simulink model "reactor"  (R2024a)
settings: Solver=ode15s  StartTime=0.0  StopTime=420*60
model workspace (MAT data in the model file):
  ratio1 = 0.5
libraries: slident x30, slpidlib x6
settings Model: Creator=kong0225  LastModifiedBy=kong0225
settings SolverCC: ZeroCrossControl=DisableAll  ZeroCrossAlgorithm=Adaptive  SolverResetMethod=Robust
settings DataIOCC: SaveState=on
settings DebuggingCC: UnconnectedInputMsg=warning  UnconnectedOutputMsg=warning  UnconnectedLineMsg=warning
settings ModelReferenceCC: EnableRefExpFcnMdlSchedulingChecks=on  ModelReferenceMinAlgLoopOccurrences=on
settings RTWCC: GPUComputeCapability=3.5  DLArmComputeVersion=19.05

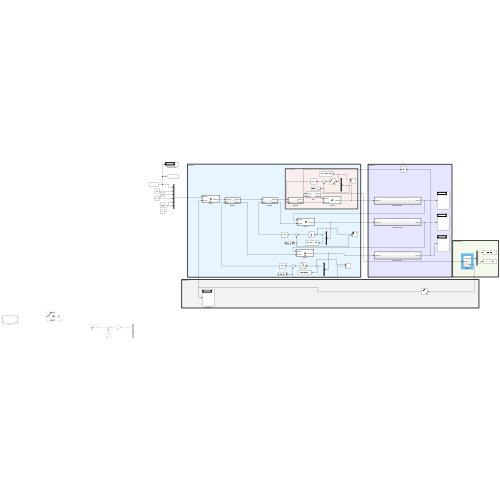
[thumbnail: Simulink's stored preview of the top-level diagram]
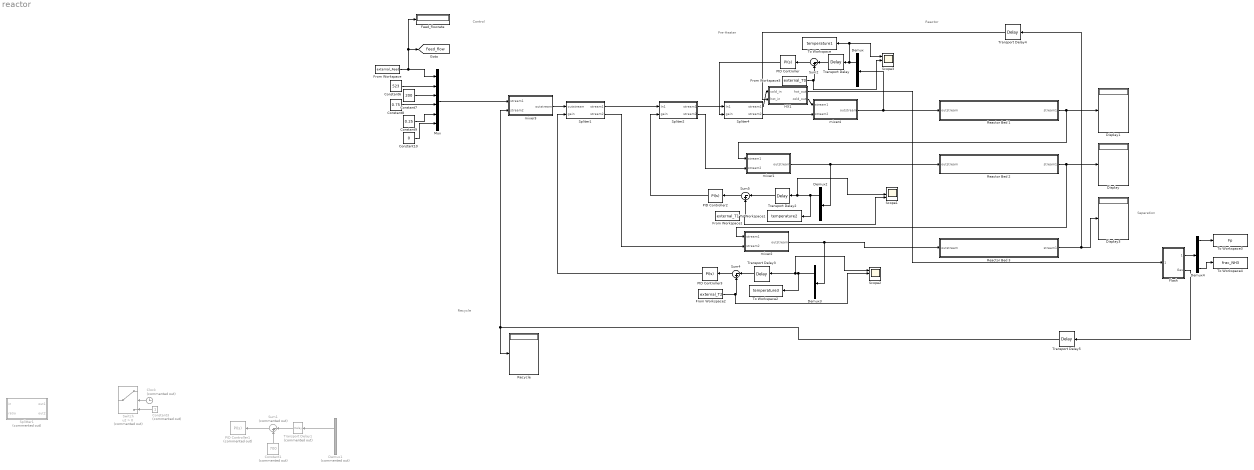
== system reactor ==
  note: Pre-Heater
  note: Control
  note: Separation
  note: Reactor
  note: Recycle
  Clock : Clock  Commented=on
  Constant1 : Constant  Commented=on  Value=700
  Constant10 : Constant  Value=0
  Constant3 : Constant  Commented=on
  Constant6 : Constant  Value=523
  Constant7 : Constant  Value=200
  Constant8 : Constant  Value=0.75
  Constant9 : Constant  Value=0.25
  Demux{,2..4} (4 alike) : Demux  Outputs=6
  Demux1 : Demux  Commented=on  Outputs=6
  Display : Display
  Display1 : Display
  Display3 : Display
  Feed_flowrate : Display
  Flash : Subsystem
  From Workspace : FromWorkspace  VariableName=external_Feed  Interpolate=off  OutputAfterFinalValue=Holding final value
  From Workspace1 : FromWorkspace  VariableName=external_T1  Interpolate=off  OutputAfterFinalValue=Holding final value
  From Workspace2 : FromWorkspace  VariableName=external_T2  Interpolate=off  OutputAfterFinalValue=Holding final value
  From Workspace3 : FromWorkspace  VariableName=external_T0  Interpolate=off  OutputAfterFinalValue=Holding final value
  HX1 : Subsystem
  Mux : Mux  Inputs=6
  PID Controller : slpidlib/PID Controller  Controller=PI  Form=Parallel  TimeDomain=Continuous-time  UseExternalTs=off  SampleTime=1  IntegratorMethod=Forward Euler  FilterMethod=Forward Euler  ControllerParametersSource=internal  P=-0.048857  I=-0.003  UseKiTs=off  D=0  UseExternalDerivativeSource=off  N=100  UseFilter=on  TunerSelectOption=Transfer Function Based (PID Tuner App)  ZeroCross=off  InitialConditionSource=internal  InitialConditionForIntegrator=0.0001  InitialConditionForFilter=0  DifferentiatorICPrevScaledInput=0  ExternalReset=none  TrackingMode=off  Kt=1  LimitOutput=off  SatLimitsSource=internal  UpperSaturationLimit=0.99  LowerSaturationLimit=-0.99  LinearizeAsGain=off  AntiWindupMode=clamping  Kb=1  LimitIntegrator=off  UpperIntegratorSaturationLimit=inf  LowerIntegratorSaturationLimit=-inf  POutMin=[]  POutMax=[]  IOutMin=[]  IOutMax=[]  DOutMin=[]  DOutMax=[]  NOutMin=[]  NOutMax=[]  SumOutMin=[]  SumOutMax=[]  SaturationOutMin=[]  SaturationOutMax=[]  PParamMin=[]  PParamMax=[]  IParamMin=[]  IParamMax=[]  DParamMin=[]  DParamMax=[]  NParamMin=[]  NParamMax=[]  KbParamMin=[]  KbParamMax=[]  KtParamMin=[]  KtParamMax=[]  KbOutMin=[]  KbOutMax=[]  KtOutMin=[]  KtOutMax=[]  IntegratorOutMin=[]  IntegratorOutMax=[]  FilterOutMin=[]  FilterOutMax=[]  SumI1OutMin=[]  SumI1OutMax=[]  SumI2OutMin=[]  SumI2OutMax=[]  SumI3OutMin=[]  SumI3OutMax=[]  SumI4OutMin=[]  SumI4OutMax=[]  SumDOutMin=[]  SumDOutMax=[]  DifferentiatorOutMin=[]  DifferentiatorOutMax=[]  FilterDiffOutCoefMin=[]  FilterDiffOutCoefMax=[]  ReciprocalOutMin=[]  ReciprocalOutMax=[]  SumDenOutMin=[]  SumDenOutMax=[]  SumNumOutMin=[]  SumNumOutMax=[]  DivideOutMin=[]  DivideOutMax=[]  UdiffTsProdOutMin=[]  UdiffTsProdOutMax=[]  NTsProdOutMin=[]  NTsProdOutMax=[]  UintegralTsProdOutMin=[]  UintegralTsProdOutMax=[]  UngainTsProdOutMin=[]  UngainTsProdOutMax=[]  ClampingZeroOutDataTypeStr=Inherit: Inherit via back propagation  ClampingZeroOutMin=[]  ClampingZeroOutMax=[]  FilterDenConstantOutDataTypeStr=Inherit: Inherit via back propagation  FilterDenConstantOutMin=[]  FilterDenConstantOutMax=[]  PCopyOutDataTypeStr=Inherit: Inherit via back propagation  PCopyOutMin=[]  PCopyOutMax=[]  NCopyOutDataTypeStr=Inherit: Inherit via back propagation  NCopyOutMin=[]  NCopyOutMax=[]  IntegratorContinuousStateAttributes=''  IntegratorStateMustResolveToSignalObject=off  IntegratorRTWStateStorageClass=Auto  FilterContinuousStateAttributes=''  FilterStateMustResolveToSignalObject=off  FilterRTWStateStorageClass=Auto  ParallelPVariant=InternalParameters  IdealPVariant=Disabled  IVariant=InternalParameters  DVariant=Disabled  IntegratorVariant=Continuous  SatVariant=Disabled  AWVariant=Passthrough  PCopyVariant=Disabled  TRVariant=Disabled  FdbkBlocksVariant=Forward  IdealPFdbkVariant=Disabled  SatFdbkVariant=Disabled  DerivativeFilterVariant=Disabled  NVariant=Disabled  NCopyVariant=Disabled_SignalSpec  FilterICVariant=Disabled  IntegratorICVariant=InternalICs  ExternalResetVariant=Disabled  TRSumVariant=Passthrough  SumFdbkVariant=Disabled  SumVariant=Sum_PI  TsampFilterVariant=InternalTs  TsampNgainVariant=Passthrough  TsampIntegralVariant=Disabled_SignalSpec  ExternalSaturationOutDataTypeStr=Inherit: Same as second input  DerivativeSourceVariant=Disabled
  PID Controller1 : slpidlib/PID Controller  Commented=on  Controller=PI  Form=Parallel  TimeDomain=Continuous-time  UseExternalTs=off  SampleTime=-1  IntegratorMethod=Forward Euler  FilterMethod=Forward Euler  ControllerParametersSource=internal  P=0.000672330279785906  I=0.00572696013263411  UseKiTs=off  D=0  UseExternalDerivativeSource=off  N=100  UseFilter=on  TunerSelectOption=Transfer Function Based (PID Tuner App)  InitialConditionSource=internal  InitialConditionForIntegrator=0  InitialConditionForFilter=0  DifferentiatorICPrevScaledInput=0  ExternalReset=none  TrackingMode=off  Kt=1  LimitOutput=on  SatLimitsSource=internal  UpperSaturationLimit=0.99  LowerSaturationLimit=0.01  LinearizeAsGain=off  AntiWindupMode=clamping  Kb=1  LimitIntegrator=off  UpperIntegratorSaturationLimit=inf  LowerIntegratorSaturationLimit=-inf  POutMin=[]  POutMax=[]  IOutMin=[]  IOutMax=[]  DOutMin=[]  DOutMax=[]  NOutMin=[]  NOutMax=[]  SumOutMin=[]  SumOutMax=[]  SaturationOutMin=[]  SaturationOutMax=[]  PParamMin=[]  PParamMax=[]  IParamMin=[]  IParamMax=[]  DParamMin=[]  DParamMax=[]  NParamMin=[]  NParamMax=[]  KbParamMin=[]  KbParamMax=[]  KtParamMin=[]  KtParamMax=[]  KbOutMin=[]  KbOutMax=[]  KtOutMin=[]  KtOutMax=[]  IntegratorOutMin=[]  IntegratorOutMax=[]  FilterOutMin=[]  FilterOutMax=[]  SumI1OutMin=[]  SumI1OutMax=[]  SumI2OutMin=[]  SumI2OutMax=[]  SumI3OutMin=[]  SumI3OutMax=[]  SumI4OutMin=[]  SumI4OutMax=[]  SumDOutMin=[]  SumDOutMax=[]  DifferentiatorOutMin=[]  DifferentiatorOutMax=[]  FilterDiffOutCoefMin=[]  FilterDiffOutCoefMax=[]  ReciprocalOutMin=[]  ReciprocalOutMax=[]  SumDenOutMin=[]  SumDenOutMax=[]  SumNumOutMin=[]  SumNumOutMax=[]  DivideOutMin=[]  DivideOutMax=[]  UdiffTsProdOutMin=[]  UdiffTsProdOutMax=[]  NTsProdOutMin=[]  NTsProdOutMax=[]  UintegralTsProdOutMin=[]  UintegralTsProdOutMax=[]  UngainTsProdOutMin=[]  UngainTsProdOutMax=[]  ClampingZeroOutDataTypeStr=Inherit: Inherit via back propagation  ClampingZeroOutMin=[]  ClampingZeroOutMax=[]  FilterDenConstantOutDataTypeStr=Inherit: Inherit via back propagation  FilterDenConstantOutMin=[]  FilterDenConstantOutMax=[]  PCopyOutDataTypeStr=Inherit: Inherit via back propagation  PCopyOutMin=[]  PCopyOutMax=[]  NCopyOutDataTypeStr=Inherit: Inherit via back propagation  NCopyOutMin=[]  NCopyOutMax=[]  IntegratorContinuousStateAttributes=''  IntegratorStateMustResolveToSignalObject=off  IntegratorRTWStateStorageClass=Auto  FilterContinuousStateAttributes=''  FilterStateMustResolveToSignalObject=off  FilterRTWStateStorageClass=Auto  ParallelPVariant=InternalParameters  IdealPVariant=Disabled  IVariant=InternalParameters  DVariant=Disabled  IntegratorVariant=Continuous  SatVariant=Enabled  AWVariant=ContClampingParallel  PCopyVariant=Disabled  TRVariant=Disabled  FdbkBlocksVariant=Forward  IdealPFdbkVariant=Disabled  SatFdbkVariant=Disabled  DerivativeFilterVariant=Disabled  NVariant=Disabled  NCopyVariant=Disabled_SignalSpec  FilterICVariant=Disabled  IntegratorICVariant=InternalICs  ExternalResetVariant=Disabled  TRSumVariant=Passthrough  SumFdbkVariant=Disabled  SumVariant=Sum_PI  TsampFilterVariant=InternalTs  TsampNgainVariant=Passthrough  TsampIntegralVariant=Passthrough  ExternalSaturationOutDataTypeStr=Inherit: Same as second input  DerivativeSourceVariant=ErrorSignal
  PID Controller2 : slpidlib/PID Controller  Controller=PI  Form=Parallel  TimeDomain=Continuous-time  UseExternalTs=off  SampleTime=1  IntegratorMethod=Forward Euler  FilterMethod=Forward Euler  ControllerParametersSource=internal  P=-0.0439115523106535  I=-0.057875624067586  UseKiTs=off  D=0  UseExternalDerivativeSource=off  N=100  UseFilter=on  TunerSelectOption=Transfer Function Based (PID Tuner App)  ZeroCross=off  InitialConditionSource=internal  InitialConditionForIntegrator=0.0001  InitialConditionForFilter=0  DifferentiatorICPrevScaledInput=0  ExternalReset=none  TrackingMode=off  Kt=1  LimitOutput=off  SatLimitsSource=internal  UpperSaturationLimit=0.99  LowerSaturationLimit=-0.99  LinearizeAsGain=off  AntiWindupMode=clamping  Kb=1  LimitIntegrator=off  UpperIntegratorSaturationLimit=inf  LowerIntegratorSaturationLimit=-inf  POutMin=[]  POutMax=[]  IOutMin=[]  IOutMax=[]  DOutMin=[]  DOutMax=[]  NOutMin=[]  NOutMax=[]  SumOutMin=[]  SumOutMax=[]  SaturationOutMin=[]  SaturationOutMax=[]  PParamMin=[]  PParamMax=[]  IParamMin=[]  IParamMax=[]  DParamMin=[]  DParamMax=[]  NParamMin=[]  NParamMax=[]  KbParamMin=[]  KbParamMax=[]  KtParamMin=[]  KtParamMax=[]  KbOutMin=[]  KbOutMax=[]  KtOutMin=[]  KtOutMax=[]  IntegratorOutMin=[]  IntegratorOutMax=[]  FilterOutMin=[]  FilterOutMax=[]  SumI1OutMin=[]  SumI1OutMax=[]  SumI2OutMin=[]  SumI2OutMax=[]  SumI3OutMin=[]  SumI3OutMax=[]  SumI4OutMin=[]  SumI4OutMax=[]  SumDOutMin=[]  SumDOutMax=[]  DifferentiatorOutMin=[]  DifferentiatorOutMax=[]  FilterDiffOutCoefMin=[]  FilterDiffOutCoefMax=[]  ReciprocalOutMin=[]  ReciprocalOutMax=[]  SumDenOutMin=[]  SumDenOutMax=[]  SumNumOutMin=[]  SumNumOutMax=[]  DivideOutMin=[]  DivideOutMax=[]  UdiffTsProdOutMin=[]  UdiffTsProdOutMax=[]  NTsProdOutMin=[]  NTsProdOutMax=[]  UintegralTsProdOutMin=[]  UintegralTsProdOutMax=[]  UngainTsProdOutMin=[]  UngainTsProdOutMax=[]  ClampingZeroOutDataTypeStr=Inherit: Inherit via back propagation  ClampingZeroOutMin=[]  ClampingZeroOutMax=[]  FilterDenConstantOutDataTypeStr=Inherit: Inherit via back propagation  FilterDenConstantOutMin=[]  FilterDenConstantOutMax=[]  PCopyOutDataTypeStr=Inherit: Inherit via back propagation  PCopyOutMin=[]  PCopyOutMax=[]  NCopyOutDataTypeStr=Inherit: Inherit via back propagation  NCopyOutMin=[]  NCopyOutMax=[]  IntegratorContinuousStateAttributes=''  IntegratorStateMustResolveToSignalObject=off  IntegratorRTWStateStorageClass=Auto  FilterContinuousStateAttributes=''  FilterStateMustResolveToSignalObject=off  FilterRTWStateStorageClass=Auto  ParallelPVariant=InternalParameters  IdealPVariant=Disabled  IVariant=InternalParameters  DVariant=Disabled  IntegratorVariant=Continuous  SatVariant=Disabled  AWVariant=Passthrough  PCopyVariant=Disabled  TRVariant=Disabled  FdbkBlocksVariant=Forward  IdealPFdbkVariant=Disabled  SatFdbkVariant=Disabled  DerivativeFilterVariant=Disabled  NVariant=Disabled  NCopyVariant=Disabled_SignalSpec  FilterICVariant=Disabled  IntegratorICVariant=InternalICs  ExternalResetVariant=Disabled  TRSumVariant=Passthrough  SumFdbkVariant=Disabled  SumVariant=Sum_PI  TsampFilterVariant=InternalTs  TsampNgainVariant=Passthrough  TsampIntegralVariant=Disabled_SignalSpec  ExternalSaturationOutDataTypeStr=Inherit: Same as second input  DerivativeSourceVariant=Disabled
  PID Controller3 : slpidlib/PID Controller  Controller=PI  Form=Parallel  TimeDomain=Continuous-time  UseExternalTs=off  SampleTime=1  IntegratorMethod=Forward Euler  FilterMethod=Forward Euler  ControllerParametersSource=internal  P=-0.021226  I=-0.00084495  UseKiTs=off  D=0  UseExternalDerivativeSource=off  N=100  UseFilter=on  TunerSelectOption=Transfer Function Based (PID Tuner App)  ZeroCross=off  InitialConditionSource=internal  InitialConditionForIntegrator=0.0001  InitialConditionForFilter=0  DifferentiatorICPrevScaledInput=0  ExternalReset=none  TrackingMode=off  Kt=1  LimitOutput=off  SatLimitsSource=internal  UpperSaturationLimit=0.99  LowerSaturationLimit=-0.99  LinearizeAsGain=off  AntiWindupMode=clamping  Kb=1  LimitIntegrator=off  UpperIntegratorSaturationLimit=inf  LowerIntegratorSaturationLimit=-inf  POutMin=[]  POutMax=[]  IOutMin=[]  IOutMax=[]  DOutMin=[]  DOutMax=[]  NOutMin=[]  NOutMax=[]  SumOutMin=[]  SumOutMax=[]  SaturationOutMin=[]  SaturationOutMax=[]  PParamMin=[]  PParamMax=[]  IParamMin=[]  IParamMax=[]  DParamMin=[]  DParamMax=[]  NParamMin=[]  NParamMax=[]  KbParamMin=[]  KbParamMax=[]  KtParamMin=[]  KtParamMax=[]  KbOutMin=[]  KbOutMax=[]  KtOutMin=[]  KtOutMax=[]  IntegratorOutMin=[]  IntegratorOutMax=[]  FilterOutMin=[]  FilterOutMax=[]  SumI1OutMin=[]  SumI1OutMax=[]  SumI2OutMin=[]  SumI2OutMax=[]  SumI3OutMin=[]  SumI3OutMax=[]  SumI4OutMin=[]  SumI4OutMax=[]  SumDOutMin=[]  SumDOutMax=[]  DifferentiatorOutMin=[]  DifferentiatorOutMax=[]  FilterDiffOutCoefMin=[]  FilterDiffOutCoefMax=[]  ReciprocalOutMin=[]  ReciprocalOutMax=[]  SumDenOutMin=[]  SumDenOutMax=[]  SumNumOutMin=[]  SumNumOutMax=[]  DivideOutMin=[]  DivideOutMax=[]  UdiffTsProdOutMin=[]  UdiffTsProdOutMax=[]  NTsProdOutMin=[]  NTsProdOutMax=[]  UintegralTsProdOutMin=[]  UintegralTsProdOutMax=[]  UngainTsProdOutMin=[]  UngainTsProdOutMax=[]  ClampingZeroOutDataTypeStr=Inherit: Inherit via back propagation  ClampingZeroOutMin=[]  ClampingZeroOutMax=[]  FilterDenConstantOutDataTypeStr=Inherit: Inherit via back propagation  FilterDenConstantOutMin=[]  FilterDenConstantOutMax=[]  PCopyOutDataTypeStr=Inherit: Inherit via back propagation  PCopyOutMin=[]  PCopyOutMax=[]  NCopyOutDataTypeStr=Inherit: Inherit via back propagation  NCopyOutMin=[]  NCopyOutMax=[]  IntegratorContinuousStateAttributes=''  IntegratorStateMustResolveToSignalObject=off  IntegratorRTWStateStorageClass=Auto  FilterContinuousStateAttributes=''  FilterStateMustResolveToSignalObject=off  FilterRTWStateStorageClass=Auto  ParallelPVariant=InternalParameters  IdealPVariant=Disabled  IVariant=InternalParameters  DVariant=Disabled  IntegratorVariant=Continuous  SatVariant=Disabled  AWVariant=Passthrough  PCopyVariant=Disabled  TRVariant=Disabled  FdbkBlocksVariant=Forward  IdealPFdbkVariant=Disabled  SatFdbkVariant=Disabled  DerivativeFilterVariant=Disabled  NVariant=Disabled  NCopyVariant=Disabled_SignalSpec  FilterICVariant=Disabled  IntegratorICVariant=InternalICs  ExternalResetVariant=Disabled  TRSumVariant=Passthrough  SumFdbkVariant=Disabled  SumVariant=Sum_PI  TsampFilterVariant=InternalTs  TsampNgainVariant=Passthrough  TsampIntegralVariant=Disabled_SignalSpec  ExternalSaturationOutDataTypeStr=Inherit: Same as second input  DerivativeSourceVariant=Disabled
  Reactor Bed 1 : Subsystem  TreatAsAtomicUnit=on
  Reactor Bed 2 : Subsystem  TreatAsAtomicUnit=on
  Reactor Bed 3 : Subsystem  TreatAsAtomicUnit=on
  Recycle : Display
  Scope1 : Scope  NumInputPorts=3
  Scope2 : Scope  NumInputPorts=3
  Scope3 : Scope  NumInputPorts=3
  Spliter1 : Subsystem  TreatAsAtomicUnit=on
  Spliter2 : Subsystem  TreatAsAtomicUnit=on
  Spliter4 : Subsystem  TreatAsAtomicUnit=on
  Splitter1 : MATLAB Function  Commented=on  TreatAsAtomicUnit=on
  Sum1 : Sum  Commented=on  Inputs=|-+
  Sum2 : Sum  Inputs=|-+
  Sum4 : Sum  Inputs=|-+
  Sum5 : Sum  Inputs=|-+
  Switch : Switch  Commented=on  Criteria=u2 > Threshold  SaturateOnIntegerOverflow=off  InputSameDT=off
  To Workspace : ToWorkspace  VariableName=temperature1  SaveFormat=Timeseries  SampleTime=-1
  To Workspace1 : ToWorkspace  VariableName=temperature2  SaveFormat=Timeseries  SampleTime=-1
  To Workspace2 : ToWorkspace  VariableName=temperature3  SaveFormat=Timeseries  SampleTime=-1
  To Workspace3 : ToWorkspace  VariableName=Fp  SaveFormat=Timeseries  SampleTime=-1
  To Workspace4 : ToWorkspace  VariableName=frac_NH3  SaveFormat=Timeseries  SampleTime=-1
  Transport Delay : TransportDelay  InitialOutput=635
  Transport Delay1 : TransportDelay  Commented=on  InitialOutput=700
  Transport Delay2 : TransportDelay  InitialOutput=635
  Transport Delay3 : TransportDelay  InitialOutput=635
  Transport Delay4 : TransportDelay  InitialOutput=[1500;726;200;0.6;0.2;0.2]
  Transport Delay5 : TransportDelay  InitialOutput=[2100;523;200;0.75;.25;0]
  mixer1 : MATLAB Function  TreatAsAtomicUnit=on
  mixer2 : MATLAB Function  TreatAsAtomicUnit=on
  mixer3 : MATLAB Function  TreatAsAtomicUnit=on
  mixer4 : MATLAB Function  TreatAsAtomicUnit=on
  tag scope: Feed_flow=global
  wires:
  Constant1/1 -> Sum1/2
  Demux1/2 -> Transport Delay1/1
  Transport Delay1/1 -> Sum1/1
  Clock/1 -> Switch/2
  Constant3/1 -> Switch/3
  Sum1/1 -> PID Controller1/1
  Constant6/1 -> Mux/2
  Constant7/1 -> Mux/3
  Constant8/1 -> Mux/4
  Constant9/1 -> Mux/5
  Constant10/1 -> Mux/6
  From Workspace/1 -> Feed_flowrate/1, [Feed_flow], Mux/1
  Demux3/2 -> Scope2/1, Transport Delay3/1, To Workspace2/1
  Demux2/2 -> Scope1/2, Transport Delay2/1, To Workspace1/1
  Flash/2(Gas) -> Transport Delay5/1
  Mux/1 -> mixer3/1(stream1)
  Spliter4/2(stream2) -> mixer4/2(stream2)
  Transport Delay3/1 -> Sum4/1
  HX1/2(cold_out) -> mixer4/1(stream1)
  Spliter2/1(stream1) -> Spliter4/1(In1)
  mixer1/1(outstream) -> Reactor Bed 2/1(outstream), Demux2/1
  Reactor Bed 1/1(stream1) -> mixer1/1(stream1), Display1/1
  mixer4/1(outstream) -> Reactor Bed 1/1(outstream), Demux/1
  From Workspace2/1 -> Scope2/2, Sum4/2
  Spliter1/2(stream2) -> mixer2/2(stream2)
  Reactor Bed 3/1(stream1) -> Transport Delay4/1, Display3/1
  Spliter2/2(stream2) -> mixer1/2(stream2)
  Spliter1/1(stream1) -> Spliter2/1(In1)
  Reactor Bed 2/1(stream1) -> mixer2/1(stream1), Display/1
  Transport Delay5/1 -> Recycle/1, mixer3/2(stream2)
  mixer2/1(outstream) -> Reactor Bed 3/1(outstream), Demux3/1
  Demux/2 -> Scope3/1, To Workspace/1, Transport Delay/1
  Transport Delay2/1 -> Sum5/1
  From Workspace1/1 -> Scope1/3, Sum5/2
  Spliter4/1(stream1) -> HX1/1(cold_in)
  From Workspace3/1 -> Scope3/2, Sum2/2
  HX1/1(hot_out) -> Flash/1(stream1)
  Flash/1(Ammonia) -> Demux4/1
  Demux4/1 -> To Workspace3/1
  Demux4/6 -> To Workspace4/1
  Transport Delay/1 -> Sum2/1
  Transport Delay4/1 -> HX1/2(hot_in)
  PID Controller/1 -> Spliter4/2(gain)
  Sum2/1 -> PID Controller/1
  PID Controller2/1 -> Spliter2/2(gain)
  Sum5/1 -> PID Controller2/1
  PID Controller3/1 -> Spliter1/2(gain)
  Sum4/1 -> PID Controller3/1
  mixer3/1(outstream) -> Spliter1/1(outstream)

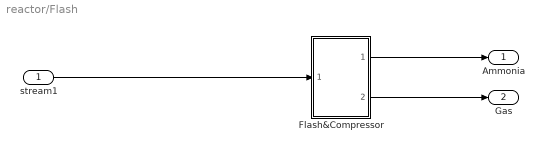
== system reactor/Flash ==
  stream1 : Inport
  Flash&Compressor : Subsystem
  Ammonia : Outport
  Gas : Outport  Port=2
  wires:
  stream1/1 -> Flash&Compressor/1(stream1)
  Flash&Compressor/1(s_prod) -> Ammonia/1
  Flash&Compressor/2(s_cyc) -> Gas/1

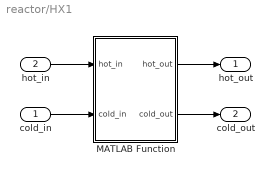
== system reactor/HX1 ==
  cold_in : Inport
  hot_in : Inport  Port=2
  MATLAB Function : MATLAB Function  TreatAsAtomicUnit=on
  hot_out : Outport
  cold_out : Outport  Port=2
  wires:
  hot_in/1 -> MATLAB Function/1(hot_in)
  cold_in/1 -> MATLAB Function/2(cold_in)
  MATLAB Function/1(hot_out) -> hot_out/1
  MATLAB Function/2(cold_out) -> cold_out/1

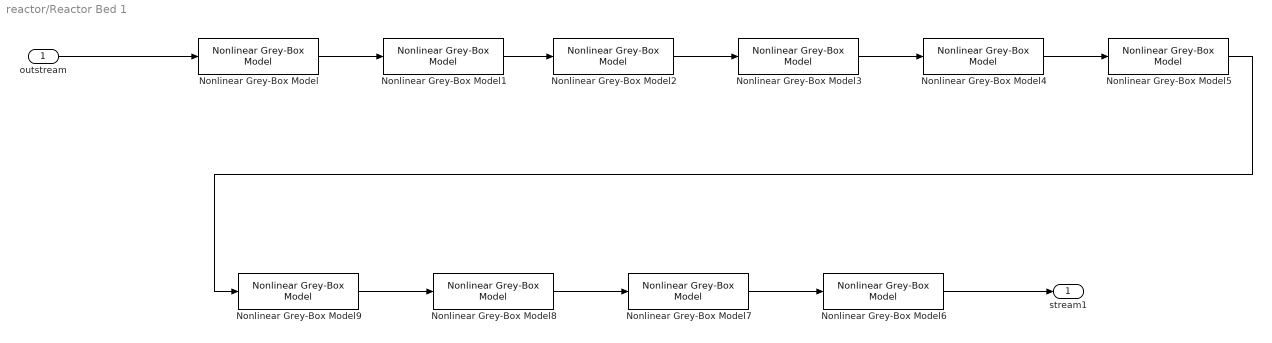
== system reactor/Reactor Bed 1 ==
  outstream : Inport
  Nonlinear Grey-Box Model : slident/Models/Nonlinear Grey-Box Model  nlsys=nlgr.nlgr_11  X0='m'
  Nonlinear Grey-Box Model1 : slident/Models/Nonlinear Grey-Box Model  nlsys=nlgr.nlgr_12  X0='m'
  Nonlinear Grey-Box Model2 : slident/Models/Nonlinear Grey-Box Model  nlsys=nlgr.nlgr_13  X0='m'
  Nonlinear Grey-Box Model3 : slident/Models/Nonlinear Grey-Box Model  nlsys=nlgr.nlgr_14  X0='m'
  Nonlinear Grey-Box Model4 : slident/Models/Nonlinear Grey-Box Model  nlsys=nlgr.nlgr_15  X0='m'
  Nonlinear Grey-Box Model5 : slident/Models/Nonlinear Grey-Box Model  nlsys=nlgr.nlgr_16  X0='m'
  Nonlinear Grey-Box Model6 : slident/Models/Nonlinear Grey-Box Model  nlsys=nlgr.nlgr_110  X0='m'
  Nonlinear Grey-Box Model7 : slident/Models/Nonlinear Grey-Box Model  nlsys=nlgr.nlgr_19  X0='m'
  Nonlinear Grey-Box Model8 : slident/Models/Nonlinear Grey-Box Model  nlsys=nlgr.nlgr_18  X0='m'
  Nonlinear Grey-Box Model9 : slident/Models/Nonlinear Grey-Box Model  nlsys=nlgr.nlgr_17  X0='m'
  stream1 : Outport
  wires:
  Nonlinear Grey-Box Model/1 -> Nonlinear Grey-Box Model1/1
  Nonlinear Grey-Box Model2/1 -> Nonlinear Grey-Box Model3/1
  Nonlinear Grey-Box Model1/1 -> Nonlinear Grey-Box Model2/1
  outstream/1 -> Nonlinear Grey-Box Model/1
  Nonlinear Grey-Box Model3/1 -> Nonlinear Grey-Box Model4/1
  Nonlinear Grey-Box Model4/1 -> Nonlinear Grey-Box Model5/1
  Nonlinear Grey-Box Model7/1 -> Nonlinear Grey-Box Model6/1
  Nonlinear Grey-Box Model8/1 -> Nonlinear Grey-Box Model7/1
  Nonlinear Grey-Box Model9/1 -> Nonlinear Grey-Box Model8/1
  Nonlinear Grey-Box Model5/1 -> Nonlinear Grey-Box Model9/1
  Nonlinear Grey-Box Model6/1 -> stream1/1

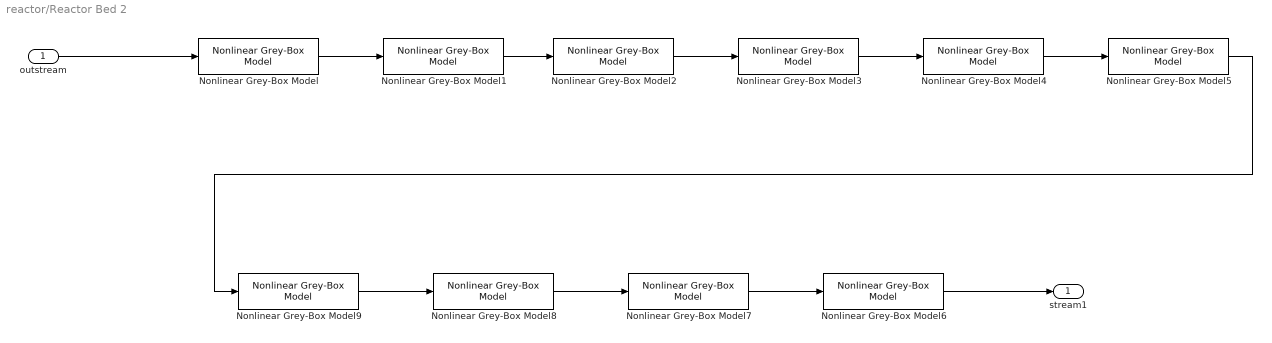
== system reactor/Reactor Bed 2 ==
  outstream : Inport
  Nonlinear Grey-Box Model : slident/Models/Nonlinear Grey-Box Model  nlsys=nlgr.nlgr_21  X0='m'
  Nonlinear Grey-Box Model1 : slident/Models/Nonlinear Grey-Box Model  nlsys=nlgr.nlgr_22  X0='m'
  Nonlinear Grey-Box Model2 : slident/Models/Nonlinear Grey-Box Model  nlsys=nlgr.nlgr_23  X0='m'
  Nonlinear Grey-Box Model3 : slident/Models/Nonlinear Grey-Box Model  nlsys=nlgr.nlgr_24  X0='m'
  Nonlinear Grey-Box Model4 : slident/Models/Nonlinear Grey-Box Model  nlsys=nlgr.nlgr_25  X0='m'
  Nonlinear Grey-Box Model5 : slident/Models/Nonlinear Grey-Box Model  nlsys=nlgr.nlgr_26  X0='m'
  Nonlinear Grey-Box Model6 : slident/Models/Nonlinear Grey-Box Model  nlsys=nlgr.nlgr_210  X0='m'
  Nonlinear Grey-Box Model7 : slident/Models/Nonlinear Grey-Box Model  nlsys=nlgr.nlgr_29  X0='m'
  Nonlinear Grey-Box Model8 : slident/Models/Nonlinear Grey-Box Model  nlsys=nlgr.nlgr_28  X0='m'
  Nonlinear Grey-Box Model9 : slident/Models/Nonlinear Grey-Box Model  nlsys=nlgr.nlgr_27  X0='m'
  stream1 : Outport
  wires:
  Nonlinear Grey-Box Model7/1 -> Nonlinear Grey-Box Model6/1
  Nonlinear Grey-Box Model9/1 -> Nonlinear Grey-Box Model8/1
  Nonlinear Grey-Box Model8/1 -> Nonlinear Grey-Box Model7/1
  Nonlinear Grey-Box Model4/1 -> Nonlinear Grey-Box Model5/1
  outstream/1 -> Nonlinear Grey-Box Model/1
  Nonlinear Grey-Box Model/1 -> Nonlinear Grey-Box Model1/1
  Nonlinear Grey-Box Model5/1 -> Nonlinear Grey-Box Model9/1
  Nonlinear Grey-Box Model1/1 -> Nonlinear Grey-Box Model2/1
  Nonlinear Grey-Box Model2/1 -> Nonlinear Grey-Box Model3/1
  Nonlinear Grey-Box Model6/1 -> stream1/1
  Nonlinear Grey-Box Model3/1 -> Nonlinear Grey-Box Model4/1

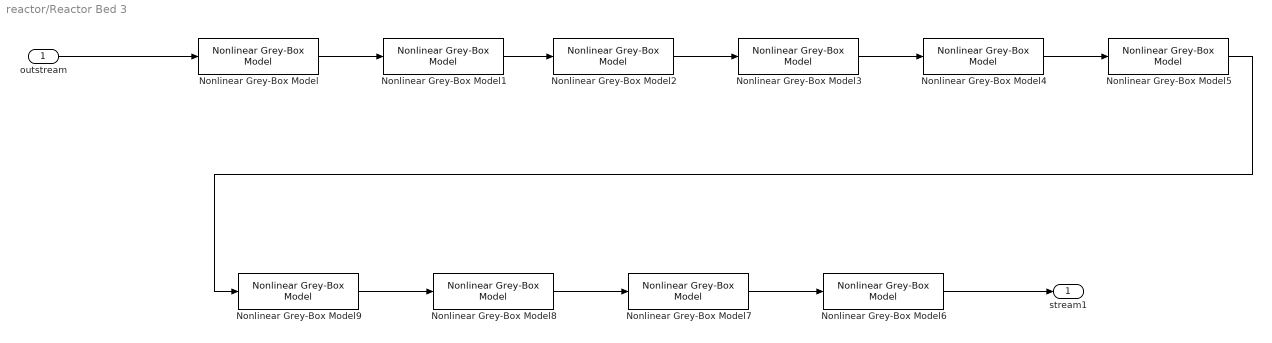
== system reactor/Reactor Bed 3 ==
  outstream : Inport
  Nonlinear Grey-Box Model : slident/Models/Nonlinear Grey-Box Model  nlsys=nlgr.nlgr_31  X0='m'
  Nonlinear Grey-Box Model1 : slident/Models/Nonlinear Grey-Box Model  nlsys=nlgr.nlgr_32  X0='m'
  Nonlinear Grey-Box Model2 : slident/Models/Nonlinear Grey-Box Model  nlsys=nlgr.nlgr_33  X0='m'
  Nonlinear Grey-Box Model3 : slident/Models/Nonlinear Grey-Box Model  nlsys=nlgr.nlgr_34  X0='m'
  Nonlinear Grey-Box Model4 : slident/Models/Nonlinear Grey-Box Model  nlsys=nlgr.nlgr_35  X0='m'
  Nonlinear Grey-Box Model5 : slident/Models/Nonlinear Grey-Box Model  nlsys=nlgr.nlgr_36  X0='m'
  Nonlinear Grey-Box Model6 : slident/Models/Nonlinear Grey-Box Model  nlsys=nlgr.nlgr_310  X0='m'
  Nonlinear Grey-Box Model7 : slident/Models/Nonlinear Grey-Box Model  nlsys=nlgr.nlgr_39  X0='m'
  Nonlinear Grey-Box Model8 : slident/Models/Nonlinear Grey-Box Model  nlsys=nlgr.nlgr_38  X0='m'
  Nonlinear Grey-Box Model9 : slident/Models/Nonlinear Grey-Box Model  nlsys=nlgr.nlgr_37  X0='m'
  stream1 : Outport
  wires:
  Nonlinear Grey-Box Model7/1 -> Nonlinear Grey-Box Model6/1
  Nonlinear Grey-Box Model9/1 -> Nonlinear Grey-Box Model8/1
  Nonlinear Grey-Box Model8/1 -> Nonlinear Grey-Box Model7/1
  Nonlinear Grey-Box Model4/1 -> Nonlinear Grey-Box Model5/1
  outstream/1 -> Nonlinear Grey-Box Model/1
  Nonlinear Grey-Box Model/1 -> Nonlinear Grey-Box Model1/1
  Nonlinear Grey-Box Model5/1 -> Nonlinear Grey-Box Model9/1
  Nonlinear Grey-Box Model1/1 -> Nonlinear Grey-Box Model2/1
  Nonlinear Grey-Box Model2/1 -> Nonlinear Grey-Box Model3/1
  Nonlinear Grey-Box Model6/1 -> stream1/1
  Nonlinear Grey-Box Model3/1 -> Nonlinear Grey-Box Model4/1

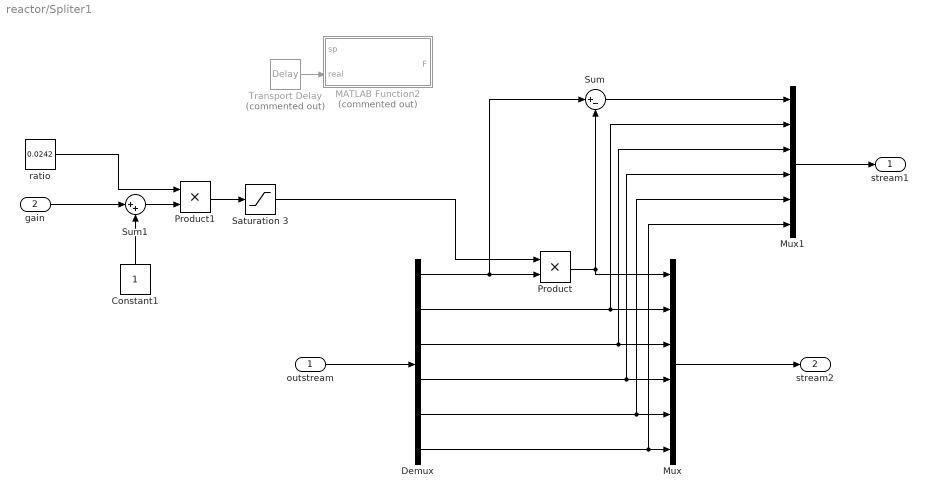
== system reactor/Spliter1 ==
  outstream : Inport
  gain : Inport  Port=2
  Constant1 : Constant
  Demux : Demux  Outputs=6
  MATLAB Function2 : MATLAB Function  Commented=on  TreatAsAtomicUnit=on
  Mux : Mux  Inputs=6
  Mux1 : Mux  Inputs=6
  Product : Product
  Product1 : Product
  Saturation 3 : Saturate  LowerLimit=0.001
  Sum : Sum  Inputs=|+-
  Sum1 : Sum  Inputs=|++
  Transport Delay : TransportDelay  Commented=on
  ratio : Constant  Value=0.0242  VectorParams1D=off
  stream1 : Outport
  stream2 : Outport  Port=2
  wires:
  outstream/1 -> Demux/1
  Demux/1 -> Sum/1, Product/2
  Product/1 -> Sum/2, Mux/1
  Demux/2 -> Mux1/2, Mux/2
  Demux/4 -> Mux1/4, Mux/4
  Demux/5 -> Mux1/5, Mux/5
  Demux/6 -> Mux1/6, Mux/6
  Sum/1 -> Mux1/1
  Demux/3 -> Mux1/3, Mux/3
  ratio/1 -> Product1/1
  gain/1 -> Sum1/1
  Constant1/1 -> Sum1/2
  Sum1/1 -> Product1/2
  Product1/1 -> Saturation 3/1
  Mux/1 -> stream2/1
  Mux1/1 -> stream1/1
  Saturation 3/1 -> Product/1
  Transport Delay/1 -> MATLAB Function2/2(real)

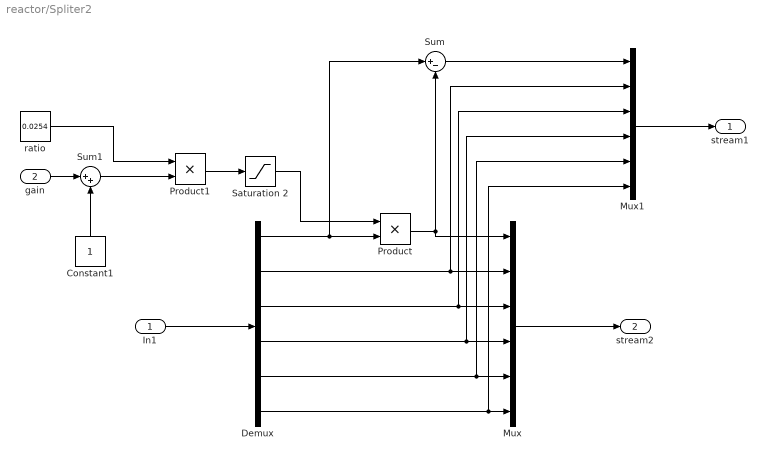
== system reactor/Spliter2 ==
  In1 : Inport
  gain : Inport  Port=2
  Constant1 : Constant
  Demux : Demux  Outputs=6
  Mux : Mux  Inputs=6
  Mux1 : Mux  Inputs=6
  Product : Product
  Product1 : Product
  Saturation 2 : Saturate  UpperLimit=0.6  LowerLimit=0.001
  Sum : Sum  Inputs=|+-
  Sum1 : Sum  Inputs=|++
  ratio : Constant  Value=0.0254
  stream1 : Outport
  stream2 : Outport  Port=2
  wires:
  In1/1 -> Demux/1
  Demux/1 -> Sum/1, Product/2
  Product/1 -> Sum/2, Mux/1
  Demux/2 -> Mux1/2, Mux/2
  Demux/4 -> Mux1/4, Mux/4
  Demux/5 -> Mux1/5, Mux/5
  Demux/6 -> Mux1/6, Mux/6
  Sum/1 -> Mux1/1
  Demux/3 -> Mux1/3, Mux/3
  Product1/1 -> Saturation 2/1
  Constant1/1 -> Sum1/2
  gain/1 -> Sum1/1
  ratio/1 -> Product1/1
  Sum1/1 -> Product1/2
  Mux/1 -> stream2/1
  Mux1/1 -> stream1/1
  Saturation 2/1 -> Product/1

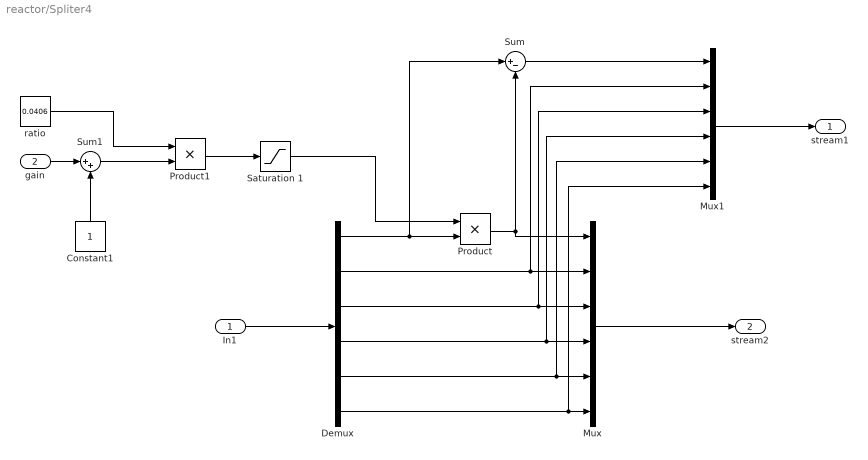
== system reactor/Spliter4 ==
  In1 : Inport
  gain : Inport  Port=2
  Constant1 : Constant
  Demux : Demux  Outputs=6
  Mux : Mux  Inputs=6
  Mux1 : Mux  Inputs=6
  Product : Product
  Product1 : Product
  Saturation 1 : Saturate  UpperLimit=0.7  LowerLimit=0.001
  Sum : Sum  Inputs=|+-
  Sum1 : Sum  Inputs=|++
  ratio : Constant  Value=0.0406
  stream1 : Outport
  stream2 : Outport  Port=2
  wires:
  In1/1 -> Demux/1
  Demux/1 -> Sum/1, Product/2
  Product/1 -> Mux/1, Sum/2
  Demux/2 -> Mux1/2, Mux/2
  Demux/4 -> Mux1/4, Mux/4
  Demux/5 -> Mux1/5, Mux/5
  Demux/6 -> Mux1/6, Mux/6
  Sum/1 -> Mux1/1
  Demux/3 -> Mux1/3, Mux/3
  Product1/1 -> Saturation 1/1
  Constant1/1 -> Sum1/2
  gain/1 -> Sum1/1
  ratio/1 -> Product1/1
  Sum1/1 -> Product1/2
  Saturation 1/1 -> Product/1
  Mux/1 -> stream2/1
  Mux1/1 -> stream1/1

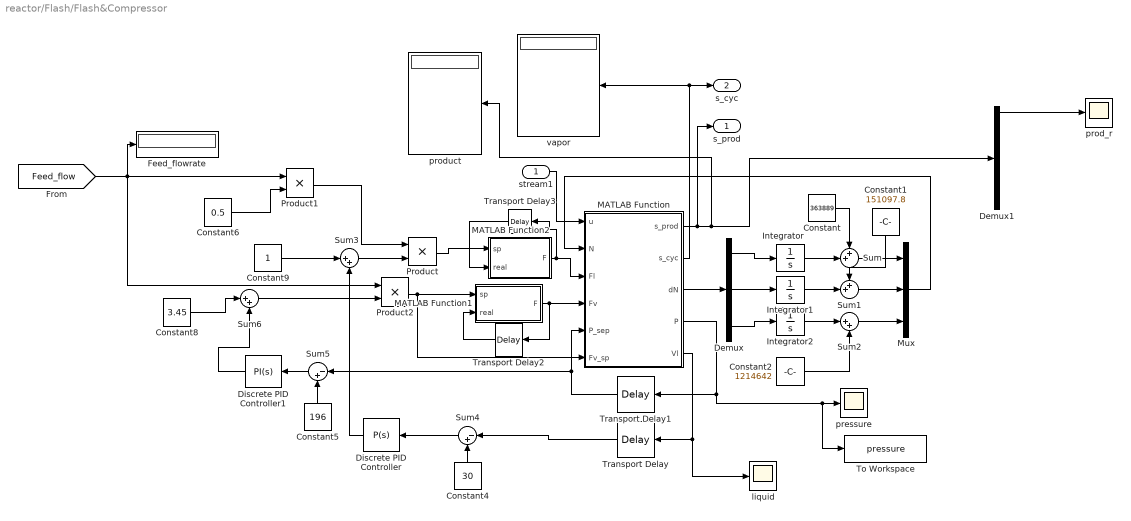
== system reactor/Flash/Flash&Compressor ==
  stream1 : Inport
  Constant : Constant  Value=363889
  Constant1 : Constant  Value=151097.8
  Constant2 : Constant  Value=1214642
  Constant4 : Constant  Value=30
  Constant5 : Constant  Value=196
  Constant6 : Constant  Value=0.5
  Constant8 : Constant  Value=3.45
  Constant9 : Constant
  Demux : Demux  Outputs=3
  Demux1 : Demux  Outputs=6
  Discrete PID Controller : slpidlib/PID Controller  Controller=P  Form=Parallel  TimeDomain=Continuous-time  UseExternalTs=off  SampleTime=-1  IntegratorMethod=Forward Euler  FilterMethod=Forward Euler  ControllerParametersSource=internal  P=-2  I=1  UseKiTs=off  D=0  UseExternalDerivativeSource=off  N=100  UseFilter=on  TunerSelectOption=Transfer Function Based (PID Tuner App)  InitialConditionSource=internal  InitialConditionForIntegrator=0  InitialConditionForFilter=0  DifferentiatorICPrevScaledInput=0  ExternalReset=none  TrackingMode=off  Kt=1  LimitOutput=on  SatLimitsSource=internal  UpperSaturationLimit=0.5  LowerSaturationLimit=-0.5  LinearizeAsGain=off  AntiWindupMode=none  Kb=1  LimitIntegrator=off  UpperIntegratorSaturationLimit=inf  LowerIntegratorSaturationLimit=-inf  POutMin=[]  POutMax=[]  IOutMin=[]  IOutMax=[]  DOutMin=[]  DOutMax=[]  NOutMin=[]  NOutMax=[]  SumOutMin=[]  SumOutMax=[]  SaturationOutMin=[]  SaturationOutMax=[]  PParamMin=[]  PParamMax=[]  IParamMin=[]  IParamMax=[]  DParamMin=[]  DParamMax=[]  NParamMin=[]  NParamMax=[]  KbParamMin=[]  KbParamMax=[]  KtParamMin=[]  KtParamMax=[]  KbOutMin=[]  KbOutMax=[]  KtOutMin=[]  KtOutMax=[]  IntegratorOutMin=[]  IntegratorOutMax=[]  FilterOutMin=[]  FilterOutMax=[]  SumI1OutMin=[]  SumI1OutMax=[]  SumI2OutMin=[]  SumI2OutMax=[]  SumI3OutMin=[]  SumI3OutMax=[]  SumI4OutMin=[]  SumI4OutMax=[]  SumDOutMin=[]  SumDOutMax=[]  DifferentiatorOutMin=[]  DifferentiatorOutMax=[]  FilterDiffOutCoefMin=[]  FilterDiffOutCoefMax=[]  ReciprocalOutMin=[]  ReciprocalOutMax=[]  SumDenOutMin=[]  SumDenOutMax=[]  SumNumOutMin=[]  SumNumOutMax=[]  DivideOutMin=[]  DivideOutMax=[]  UdiffTsProdOutMin=[]  UdiffTsProdOutMax=[]  NTsProdOutMin=[]  NTsProdOutMax=[]  UintegralTsProdOutMin=[]  UintegralTsProdOutMax=[]  UngainTsProdOutMin=[]  UngainTsProdOutMax=[]  ClampingZeroOutDataTypeStr=Inherit: Inherit via back propagation  ClampingZeroOutMin=[]  ClampingZeroOutMax=[]  FilterDenConstantOutDataTypeStr=Inherit: Inherit via back propagation  FilterDenConstantOutMin=[]  FilterDenConstantOutMax=[]  PCopyOutDataTypeStr=Inherit: Inherit via back propagation  PCopyOutMin=[]  PCopyOutMax=[]  NCopyOutDataTypeStr=Inherit: Inherit via back propagation  NCopyOutMin=[]  NCopyOutMax=[]  IntegratorContinuousStateAttributes=''  IntegratorStateMustResolveToSignalObject=off  IntegratorRTWStateStorageClass=Auto  FilterContinuousStateAttributes=''  FilterStateMustResolveToSignalObject=off  FilterRTWStateStorageClass=Auto  ParallelPVariant=InternalParameters  IdealPVariant=Disabled  IVariant=Disabled  DVariant=Disabled  IntegratorVariant=Disabled  SatVariant=Enabled  AWVariant=Disabled  PCopyVariant=Disabled  TRVariant=Disabled  FdbkBlocksVariant=Forward  IdealPFdbkVariant=Disabled  SatFdbkVariant=Disabled  DerivativeFilterVariant=Disabled  NVariant=Disabled  NCopyVariant=Disabled_SignalSpec  FilterICVariant=Disabled  IntegratorICVariant=Disabled  ExternalResetVariant=Disabled  TRSumVariant=Passthrough  SumFdbkVariant=Disabled  SumVariant=Passthrough_P  TsampFilterVariant=InternalTs  TsampNgainVariant=Passthrough  TsampIntegralVariant=Disabled_SignalSpec  ExternalSaturationOutDataTypeStr=Inherit: Same as second input  DerivativeSourceVariant=Disabled
  Discrete PID Controller1 : slpidlib/PID Controller  Controller=PI  Form=Parallel  TimeDomain=Continuous-time  UseExternalTs=off  SampleTime=-1  IntegratorMethod=Forward Euler  FilterMethod=Forward Euler  ControllerParametersSource=internal  P=-0.254  I=-0.0003  UseKiTs=off  D=-417.104440098683  UseExternalDerivativeSource=off  N=0.0199591173186702  UseFilter=on  TunerSelectOption=Transfer Function Based (PID Tuner App)  InitialConditionSource=internal  InitialConditionForIntegrator=0  InitialConditionForFilter=0  DifferentiatorICPrevScaledInput=0  ExternalReset=none  TrackingMode=off  Kt=1  LimitOutput=on  SatLimitsSource=internal  UpperSaturationLimit=1.5  LowerSaturationLimit=-1.5  LinearizeAsGain=on  AntiWindupMode=none  Kb=1  LimitIntegrator=off  UpperIntegratorSaturationLimit=inf  LowerIntegratorSaturationLimit=-inf  POutMin=[]  POutMax=[]  IOutMin=[]  IOutMax=[]  DOutMin=[]  DOutMax=[]  NOutMin=[]  NOutMax=[]  SumOutMin=[]  SumOutMax=[]  SaturationOutMin=[]  SaturationOutMax=[]  PParamMin=[]  PParamMax=[]  IParamMin=[]  IParamMax=[]  DParamMin=[]  DParamMax=[]  NParamMin=[]  NParamMax=[]  KbParamMin=[]  KbParamMax=[]  KtParamMin=[]  KtParamMax=[]  KbOutMin=[]  KbOutMax=[]  KtOutMin=[]  KtOutMax=[]  IntegratorOutMin=[]  IntegratorOutMax=[]  FilterOutMin=[]  FilterOutMax=[]  SumI1OutMin=[]  SumI1OutMax=[]  SumI2OutMin=[]  SumI2OutMax=[]  SumI3OutMin=[]  SumI3OutMax=[]  SumI4OutMin=[]  SumI4OutMax=[]  SumDOutMin=[]  SumDOutMax=[]  DifferentiatorOutMin=[]  DifferentiatorOutMax=[]  FilterDiffOutCoefMin=[]  FilterDiffOutCoefMax=[]  ReciprocalOutMin=[]  ReciprocalOutMax=[]  SumDenOutMin=[]  SumDenOutMax=[]  SumNumOutMin=[]  SumNumOutMax=[]  DivideOutMin=[]  DivideOutMax=[]  UdiffTsProdOutMin=[]  UdiffTsProdOutMax=[]  NTsProdOutMin=[]  NTsProdOutMax=[]  UintegralTsProdOutMin=[]  UintegralTsProdOutMax=[]  UngainTsProdOutMin=[]  UngainTsProdOutMax=[]  ClampingZeroOutDataTypeStr=Inherit: Inherit via back propagation  ClampingZeroOutMin=[]  ClampingZeroOutMax=[]  FilterDenConstantOutDataTypeStr=Inherit: Inherit via back propagation  FilterDenConstantOutMin=[]  FilterDenConstantOutMax=[]  PCopyOutDataTypeStr=Inherit: Inherit via back propagation  PCopyOutMin=[]  PCopyOutMax=[]  NCopyOutDataTypeStr=Inherit: Inherit via back propagation  NCopyOutMin=[]  NCopyOutMax=[]  IntegratorContinuousStateAttributes=''  IntegratorStateMustResolveToSignalObject=off  IntegratorRTWStateStorageClass=Auto  FilterContinuousStateAttributes=''  FilterStateMustResolveToSignalObject=off  FilterRTWStateStorageClass=Auto  ParallelPVariant=InternalParameters  IdealPVariant=Disabled  IVariant=InternalParameters  DVariant=Disabled  IntegratorVariant=Continuous  SatVariant=Enabled  AWVariant=Passthrough  PCopyVariant=Disabled  TRVariant=Disabled  FdbkBlocksVariant=Forward  IdealPFdbkVariant=Disabled  SatFdbkVariant=Disabled  DerivativeFilterVariant=Disabled  NVariant=Disabled  NCopyVariant=Disabled_SignalSpec  FilterICVariant=Disabled  IntegratorICVariant=InternalICs  ExternalResetVariant=Disabled  TRSumVariant=Passthrough  SumFdbkVariant=Disabled  SumVariant=Sum_PI  TsampFilterVariant=InternalTs  TsampNgainVariant=Passthrough  TsampIntegralVariant=Disabled_SignalSpec  ExternalSaturationOutDataTypeStr=Inherit: Same as second input  DerivativeSourceVariant=Disabled
  Feed_flowrate : Display
  Integrator : Integrator
  Integrator1 : Integrator
  Integrator2 : Integrator
  MATLAB Function : MATLAB Function  TreatAsAtomicUnit=on
  MATLAB Function1 : MATLAB Function  TreatAsAtomicUnit=on
  MATLAB Function2 : MATLAB Function  TreatAsAtomicUnit=on
  Mux : Mux  Inputs=3
  Product : Product
  Product1 : Product
  Product2 : Product
  Sum : Sum  Inputs=++|
  Sum1 : Sum  Inputs=++|
  Sum2 : Sum  Inputs=|++
  Sum3 : Sum  Inputs=|++
  Sum4 : Sum  Inputs=|-+
  Sum5 : Sum  Inputs=|-+
  Sum6 : Sum  Inputs=|++
  To Workspace : ToWorkspace  VariableName=pressure  SaveFormat=Timeseries  SampleTime=-1
  Transport Delay : TransportDelay  InitialOutput=30
  Transport Delay1 : TransportDelay  InitialOutput=196
  Transport Delay2 : TransportDelay  DelayTime=10  InitialOutput=1045
  Transport Delay3 : TransportDelay  DelayTime=10  InitialOutput=152
  liquid : Scope
  pressure : Scope
  prod_r : Scope
  product : Display
  vapor : Display
  s_prod : Outport
  s_cyc : Outport  Port=2
  wires:
  stream1/1 -> MATLAB Function/1(u)
  MATLAB Function/3(dN) -> Demux/1
  Demux/1 -> Integrator/1
  Demux/2 -> Integrator1/1
  Demux/3 -> Integrator2/1
  Integrator/1 -> Sum/2
  Constant/1 -> Sum/1
  Integrator1/1 -> Sum1/2
  Constant1/1 -> Sum1/1
  Integrator2/1 -> Sum2/1
  Constant2/1 -> Sum2/2
  Sum1/1 -> Mux/2
  Sum/1 -> Mux/1
  Sum2/1 -> Mux/3
  MATLAB Function/4(P) -> To Workspace/1, pressure/1, Transport Delay1/1
  Transport Delay1/1 -> Sum5/1, MATLAB Function/5(P_sep)
  MATLAB Function/1(s_prod) -> product/1, Demux1/1, s_prod/1
  MATLAB Function/2(s_cyc) -> s_cyc/1, vapor/1
  MATLAB Function/5(Vl) -> liquid/1, Transport Delay/1
  Sum4/1 -> Discrete PID Controller/1
  Constant4/1 -> Sum4/2
  Constant5/1 -> Sum5/2
  Transport Delay/1 -> Sum4/1
  Discrete PID Controller/1 -> Sum3/2
  Constant9/1 -> Sum3/1
  Sum3/1 -> Product/2
  Product1/1 -> Product/1
  Mux/1 -> MATLAB Function/2(N)
  Sum5/1 -> Discrete PID Controller1/1
  Product2/1 -> MATLAB Function/6(Fv_sp), MATLAB Function1/1(sp)
  Discrete PID Controller1/1 -> Sum6/2
  Constant8/1 -> Sum6/1
  Sum6/1 -> Product2/2
  Constant6/1 -> Product1/2
  MATLAB Function1/1(F) -> Transport Delay2/1, MATLAB Function/4(Fv)
  Transport Delay2/1 -> MATLAB Function1/2(real)
  MATLAB Function2/1(F) -> MATLAB Function/3(Fl), Transport Delay3/1
  Transport Delay3/1 -> MATLAB Function2/2(real)
  Product/1 -> MATLAB Function2/1(sp)
  [Feed_flow] -> Product2/1, Feed_flowrate/1, Product1/1
  Demux1/1 -> prod_r/1

== matlab function reactor/mixer4 ==
  data: stream1 input; outstream output; stream2 input
function outstream = mix(stream1,stream2)

T1 = stream1(2);
T2 = stream2(2);
F1 = stream1(1);
F2 = stream2(1);
CP1 = Cp(T1,stream1(3),stream1(4:6));
CP2 = Cp(T2,stream2(3),stream2(4:6));
F = F1+F2;
T = (F1*CP1*T1+F2*CP2*T2)/(F1*CP1+F2*CP2);
P = max([stream1(3),stream2(3)]);
z1 = (F1*stream1(4)+F2*stream2(4))/(F1+F2);
z2 = (F1*stream1(5)+F2*stream2(5))/(F1+F2);
z3 = (F1*stream1(6)+F2*stream2(6))/(F1+F2);
outstream = [F;T;P;z1;z2;z3];

== matlab function reactor/Flash/Flash&Compressor/MATLAB Function ==
  data: u input; s_prod output size=6; N input size=3; Fl input size=1; Fv input size=1; s_cyc output size=6; dN output; P_sep input size=1; P output size=1; Vl output size=1; Fv_sp input size=1
function [s_prod, s_cyc, dN, P, Vl] = sep_cal(u, N, Fl, Fv, P_sep, Fv_sp)
dN = zeros(length(N),1);
T_sep = 313;
%P_sep = 196;
V_sep = 100;
f = @(X) VLE(X,T_sep,P_sep,N);
options = optimoptions('fsolve','Algorithm','levenberg-marquardt','Display','off');
x0 = [0.527229,1.202400,0.69,0.23,0.076,0.02,0.005,0.975];
sol = fsolve(f, x0, options);
%sol = VLE_constr(T_sep,P_sep,N);
Nv = sol(1);
Nl = sol(2);
z_v = sol(3:5);
z_l = sol(6:8);
for i = 1:length(N)
    dN(i) = u(1)*u(i+3) - Fl*z_l(i) - max([Fv,Fv_sp])*z_v(i);
end
s_cyc = [Fv;523; 200; z_v(1) ;z_v(2); z_v(3)];
s_prod = [Fl ;T_sep; P_sep;z_l(1) ;z_l(2) ;z_l(3)];
Vl = Nl/0.04008;
P = Nv/1e-1/(V_sep-Vl)*8.314*T_sep;

== matlab function reactor/mixer1 ==
  data: stream1 input; outstream output; stream2 input
function outstream = mix(stream1,stream2)


T1 = stream1(2);
T2 = stream2(2);
F1 = stream1(1);
F2 = stream2(1);
CP1 = Cp(T1,stream1(3),stream1(4:6));
CP2 = Cp(T2,stream2(3),stream2(4:6));
F = F1+F2;
T = (F1*CP1*T1+F2*CP2*T2)/(F1*CP1+F2*CP2);
P = max([stream1(3),stream2(3)]);
z1 = (F1*stream1(4)+F2*stream2(4))/(F1+F2);
z2 = (F1*stream1(5)+F2*stream2(5))/(F1+F2);
z3 = (F1*stream1(6)+F2*stream2(6))/(F1+F2);
outstream = [F;T;P;z1;z2;z3];

== matlab function reactor/Splitter1 ==
  data: in input; out1 output; ratio input; out2 output
function [out1,out2] = spliter(in, ratio)
coeff1 = ones(6,1);
coeff2 = ones(6,1);
coeff1(1) = ratio;
coeff2(1) = 1 - ratio;
out1 = in.*coeff1;
out2 = in.*coeff2;

== matlab function reactor/mixer2 ==
  data: stream1 input; outstream output; stream2 input
function outstream = mix(stream1,stream2)


T1 = stream1(2);
T2 = stream2(2);
F1 = stream1(1);
F2 = stream2(1);
CP1 = Cp(T1,stream1(3),stream1(4:6));
CP2 = Cp(T2,stream2(3),stream2(4:6));
F = F1+F2;
T = (F1*CP1*T1+F2*CP2*T2)/(F1*CP1+F2*CP2);
P = max([stream1(3),stream2(3)]);
z1 = (F1*stream1(4)+F2*stream2(4))/(F1+F2);
z2 = (F1*stream1(5)+F2*stream2(5))/(F1+F2);
z3 = (F1*stream1(6)+F2*stream2(6))/(F1+F2);
outstream = [F;T;P;z1;z2;z3];

== matlab function reactor/HX1/MATLAB Function ==
  data: hot_in input size=6; hot_out output size=6; cold_in input size=6; cold_out output size=6
function [hot_out, cold_out] = HX(hot_in, cold_in)
U = 536;
A = 180;
Cmin = min([hot_in(1)*Cp(hot_in(2),hot_in(3),hot_in(4:6)), cold_in(1)*Cp(cold_in(2),cold_in(3),cold_in(4:6))]);
Cmax = max([hot_in(1)*Cp(hot_in(2),hot_in(3),hot_in(4:6)), cold_in(1)*Cp(cold_in(2),cold_in(3),cold_in(4:6))]);
Cr = Cmin/Cmax;
qmax = Cmin*(hot_in(2)-cold_in(2));
NTU = U*A/Cmin;
if Cr == 1
    %eps = NTU/(1+NTU);
    eps = (1-exp(-NTU*(1-Cr)))/(1-Cr*exp(-NTU*(1-Cr)));
else
    eps = (1-exp(-NTU*(1-Cr)))/(1-Cr*exp(-NTU*(1-Cr)));
end
q = qmax*eps;
Tco = q/(cold_in(1)*Cp(cold_in(2),cold_in(3),cold_in(4:6))) + cold_in(2);
Tho = -q/(hot_in(1)*Cp(hot_in(2),hot_in(3),hot_in(4:6))) + hot_in(2);
hot_out = [hot_in(1) ;Tho ;hot_in(3); hot_in(4); hot_in(5) ;hot_in(6)];
cold_out = [cold_in(1); Tco; cold_in(3); cold_in(4) ;cold_in(5) ;cold_in(6)];

== matlab function reactor/Flash/Flash&Compressor/MATLAB Function1 ==
  data: sp input; F output; real input
function F = valve(sp,real)
if sp > real
    F = real + min(0.1*real, (sp - real));
elseif sp < real
    F = real - min(0.1*real, (real-sp));
else
    F = real;
end

== matlab function reactor/mixer3 ==
  data: stream1 input; outstream output; stream2 input
function outstream = mix(stream1,stream2)


T1 = stream1(2);
T2 = stream2(2);
F1 = stream1(1);
F2 = stream2(1);
CP1 = Cp(T1,stream1(3),stream1(4:6));
CP2 = Cp(T2,stream2(3),stream2(4:6));
F = F1+F2;
T = (F1*CP1*T1+F2*CP2*T2)/(F1*CP1+F2*CP2);
P = max([stream1(3),stream2(3)]);
z1 = (F1*stream1(4)+F2*stream2(4))/(F1+F2);
z2 = (F1*stream1(5)+F2*stream2(5))/(F1+F2);
z3 = (F1*stream1(6)+F2*stream2(6))/(F1+F2);
outstream = [F;T;P;z1;z2;z3];

== matlab function reactor/Flash/Flash&Compressor/MATLAB Function2 ==
  data: sp input; F output; real input
function F = valve(sp,real)
if sp > real
    F = real + min(0.1*real, (sp - real));
elseif sp < real
    F = real - min(0.1*real, (real-sp));
else
    F = real;
end

== matlab function reactor/Spliter1/MATLAB Function2 ==
  data: sp input; F output; real input
function F = valve_feed(sp,real)
if sp > real
    F = real + min(0.2, (sp - real));
elseif sp < real
    F = real - min(0.2, (real-sp));
else
    F = real;
end
